simulink model "P4p2_integral"  (R2014a)
settings: Solver=ode1  StartTime=0.0  StopTime=inf  FixedStep=0.002  RelTol=1e-3
PostLoadFcn:
  | qc_set_target_type(getConfigSet(bdroot, 'QUARC Default Target Configuration'));
values from neighbouring files (symbols this model uses):
  A_est = [0 1 0 0 0 0; 0 0 0 0 0 0; 0 0 0 1 0 0; 0 0 0 0 0 0; 0 0 0 0 0 1; k_3 0 0 0 0 0]    [P4p2_init.m]    (also in P4p2_integral_init.m = [0 1 0 0 0 0; 0 0 0 0 0 0; 0 0 0 1 0 0; P4p3_init.m = [0 1 0 0 0 0; 0 0 0 0 0 0; 0 0 0 1 0 0)
  B_est = [0 0; 0 k_1; 0 0; k_2 0;0 0; 0 0]    [P4p2_init.m]    (also in P4p2_integral_init.m; P4p3_init.m)
  C_est = [1 0 0 0 0 0; 0 0 1 0 0 0; 0 0 0 0 1 0]    [P4p2_init.m]    (also in P4p2_integral_init.m; P4p3_init.m = [0 0 1 0 0 0; 0 0 0 0 1 0])
  Joystick_gain_x = 1    [P4p2_init.m]    (also in P4p2_integral_init.m; P4p3_init.m)
  Joystick_gain_y = -1    [P4p2_init.m]    (also in P4p2_integral_init.m; P4p3_init.m)
  K = lqr(A, B, Q, R)    [P4p2_init.m]    (also in P4p2_integral_init.m = lqr(A,B,Q,R); P4p3_init.m = lqr(A,B,Q,R))
  L = (place(A_est', C_est', poles)')    [P4p2_init.m]    (also in P4p2_integral_init.m; P4p3_init.m)
  P = inv(C*(inv(B*K - A))*B)    [P4p2_init.m]    (also in P4p2_integral_init.m = [0  K(2,1); K(1,3) 0]; P4p3_init.m = [0  K(2,1); K(1,3) 0])
  v_star = 6.8    [P4p2_init.m]    (also in P4p2_integral_init.m; P4p3_init.m)
undefined symbols (not defined in the file or in its folder): HIL, qc_get_step_size
libraries: simulink_extras x7, quarc_library x4
settings Model: SimulationMode=external  ExtModeTrigDuration=5000  Creator=Rchan  LastModifiedBy=kajajs
settings SolverCC: PositivePriorityOrder=on
settings DataIOCC: SignalLoggingSaveFormat=ModelDataLogs
settings OptimizationCC: ExpressionDepthLimit=2147483647  InitFltsAndDblsToZero=on
settings DebuggingCC: SaveWithParameterizedLinksMsg=none  UnderspecifiedInitializationDetection=Classic  MultiTaskDSMMsg=warning  MultiTaskCondExecSysMsg=none  FcnCallInpInsideContextMsg=UseLocalSettings  StateNameClashWarn=warning
settings RTWCC: SystemTargetFile=quarc_win64.tlc  TemplateMakefile=quarc_default_tmf  Description=QUARC Win64 Target  ProcessScript=quarc_win64_make_rtw_hook
settings STFCustomTargetCC: CPPClassGenCompliant=on
settings GRTTargetCC: ParMdlRefBuildCompliant=off  CompOptLevelCompliant=off  CombineOutputUpdateFcns=off  MatFileLogging=off  GRTInterface=on  ExtMode=on  ExtModeMexFile=quarc_comm

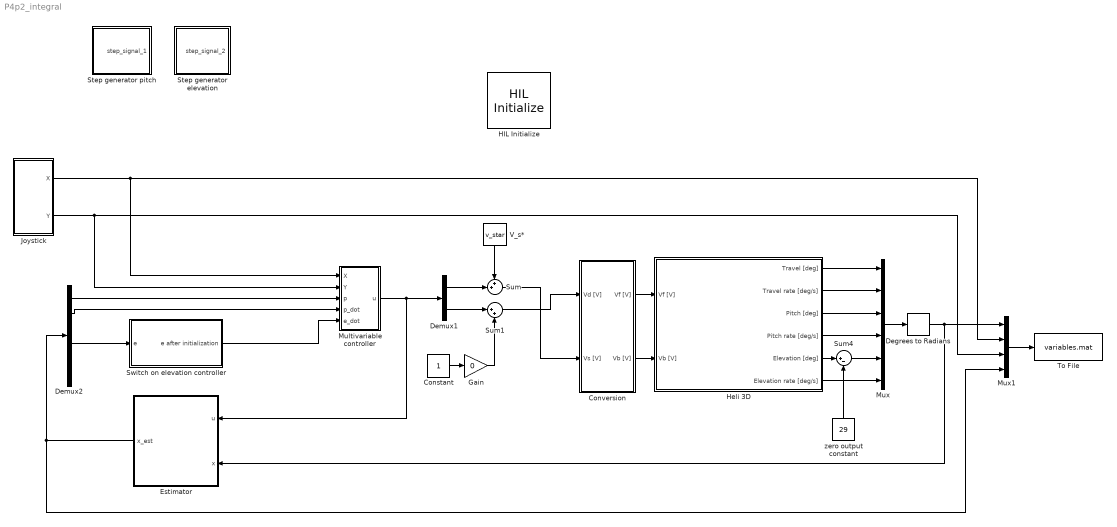
== system P4p2_integral ==
  " Switch on elevation controller" : Subsystem
  Constant : Constant
  Conversion : Subsystem
  Degrees to Radians : simulink_extras/Transformations/Degrees to Radians
  Demux1 : Demux  Outputs=2
  Demux2 : Demux  Outputs=6
  Estimator : Subsystem
  Gain : Gain  Gain=0
  HIL Initialize : quarc_library/Data Acquisition/Generic/Configuration/HIL Initialize  Priority=-99  object_name=HIL-1  board_type=q8_usb  board_number=0  board_options=update_rate=normal;decimation=1  exclusive=off  active=off  hardware_clocks=[0:2]  clock_modes=[]  initial_clock_frequencies=[]  set_clock_params_at_start=off  set_clock_params_at_switch_in=off  set_clock_frequencies_at_start=off  set_clock_frequencies_at_switch_in=off  analog_input_channels=[0:7]  analog_input_maximums=10  analog_input_minimums=-10  set_analog_input_params_at_start=on  set_analog_input_params_at_switch_in=off  analog_output_channels=[0:7]  analog_output_maximums=10  analog_output_minimums=-10  initial_analog_outputs=[0]  final_analog_outputs=[0]  watchdog_analog_outputs=0  set_analog_output_params_at_start=on  set_analog_output_params_at_switch_in=off  set_analog_outputs_at_start=on  set_analog_outputs_at_switch_in=off  set_analog_outputs_at_terminate=on  set_analog_outputs_at_switch_out=off  set_analog_outputs_on_watchdog=off  digital_input_channels=[]  digital_output_channels=[]  digital_output_configuration=[]  initial_digital_outputs=[1]  final_digital_outputs=[1]  watchdog_digital_outputs=[1]  set_digital_output_params_at_start=off  set_digital_output_params_at_switch_in=off  set_digital_outputs_at_start=on  set_digital_outputs_at_switch_in=off  set_digital_outputs_at_terminate=on  set_digital_outputs_at_switch_out=off  set_digital_outputs_on_watchdog=off  encoder_channels=[0:7]  quadrature=[4]  encoder_filter_frequency=[]  initial_encoder_counts=[0]  set_encoder_params_at_start=on  set_encoder_params_at_switch_in=off  set_encoder_counts_at_start=on  set_encoder_counts_at_switch_in=off  pwm_channels=[0:7]  pwm_modes=0  pwm_frequency=99.532799999999995e6/4095  pwm_configuration=[0]  pwm_alignment=[0]  pwm_polarity=[1]  pwm_leading_deadband=[0]  pwm_trailing_deadband=[0]  initial_pwm_outputs=[0]  final_pwm_outputs=[0]  watchdog_pwm_outputs=[0]  set_pwm_params_at_start=on  set_pwm_params_at_switch_in=off  set_pwm_outputs_at_start=on  set_pwm_outputs_at_switch_in=off  set_pwm_outputs_at_terminate=on  set_pwm_outputs_at_switch_out=off  set_pwm_outputs_on_watchdog=off  other_output_channels=[]  initial_other_outputs=[]  final_other_outputs=[]  watchdog_other_outputs=[]  set_other_outputs_at_start=off  set_other_outputs_at_switch_in=off  set_other_outputs_at_terminate=off  set_other_outputs_at_switch_out=off  set_other_outputs_on_watchdog=off
  Heli 3D : Subsystem
  Joystick : Subsystem
  "Multivariable controller " : Subsystem
  Mux : Mux  Inputs=6
  Mux1 : Mux
  Step generator elevation : Subsystem
  Step generator pitch : Subsystem
  Sum : Sum  Inputs=++|
  Sum1 : Sum  Inputs=|++
  Sum4 : Sum  Inputs=|+-
  To File : ToFile  Filename=variables.mat  MatrixName=variables
  "V_s*    " : Constant  Value=v_star
  zero output constant : Constant  Value=29
  wires:
  Conversion/2(Vb [V]) -> Heli 3D/2(Vb [V])
  Conversion/1(Vf [V]) -> Heli 3D/1(Vf [V])
  Heli 3D/1(Travel [deg]) -> Mux/1
  Heli 3D/2(Travel rate [deg/s]) -> Mux/2
  Heli 3D/4(Pitch rate [deg/s]) -> Mux/4
  Heli 3D/6(Elevation rate [deg/s]) -> Mux/6
  "Multivariable controller "/1(u) -> Estimator/1(u), Demux1/1
  Mux/1 -> Degrees to Radians/1
  Degrees to Radians/1 -> Mux1/1, Estimator/2(x)
  Sum/1 -> Conversion/2(Vs [V])
  Mux1/1 -> To File/1
  Demux1/2 -> Sum1/1
  Sum1/1 -> Conversion/1(Vd [V])
  Constant/1 -> Gain/1
  Gain/1 -> Sum1/2
  Joystick/1(X) -> Mux1/2, "Multivariable controller "/1(X)
  Joystick/2(Y) -> Mux1/3, "Multivariable controller "/2(Y)
  Demux1/1 -> Sum/2
  Heli 3D/5(Elevation [deg]) -> Sum4/1
  Sum4/1 -> Mux/5
  zero output constant/1 -> Sum4/2
  Heli 3D/3(Pitch [deg]) -> Mux/3
  "V_s*    "/1 -> Sum/1
  Estimator/1(x_est) -> Mux1/4, Demux2/1
  " Switch on elevation controller"/1("e after initialization ") -> "Multivariable controller "/5(e_dot)
  Demux2/4 -> " Switch on elevation controller"/1(e)
  Demux2/1 -> "Multivariable controller "/3(p)
  Demux2/2 -> "Multivariable controller "/4(p_dot)

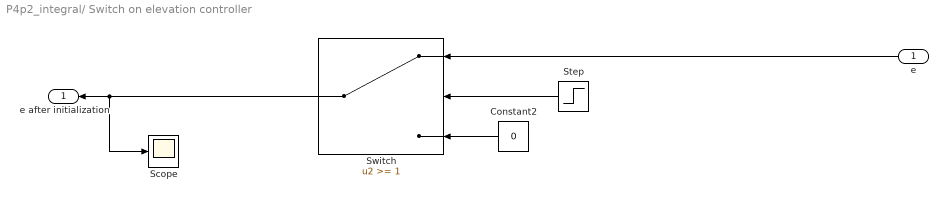
== system P4p2_integral/ Switch on elevation controller ==
  e : Inport
  Constant2 : Constant  Value=0
  Scope : Scope
      settings: YMin=-2.25  YMax=2
  Step : Step  Time=5  SampleTime=0
  Switch : Switch  Threshold=1
  "e after initialization " : Outport
  wires:
  Switch/1 -> Scope/1, "e after initialization "/1
  Constant2/1 -> Switch/3
  e/1 -> Switch/1
  Step/1 -> Switch/2

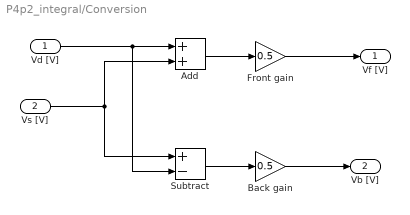
== system P4p2_integral/Conversion ==
  Vd [V] : Inport
  Vs [V] : Inport  Port=2
  Add : Sum
  Back gain : Gain  Gain=0.5
  Front gain : Gain  Gain=0.5
  Subtract : Sum  Inputs=+-
  Vf [V] : Outport
  Vb [V] : Outport  Port=2
  wires:
  Vd [V]/1 -> Subtract/2, Add/1
  Vs [V]/1 -> Subtract/1, Add/2
  Subtract/1 -> Back gain/1
  Back gain/1 -> Vb [V]/1
  Add/1 -> Front gain/1
  Front gain/1 -> Vf [V]/1

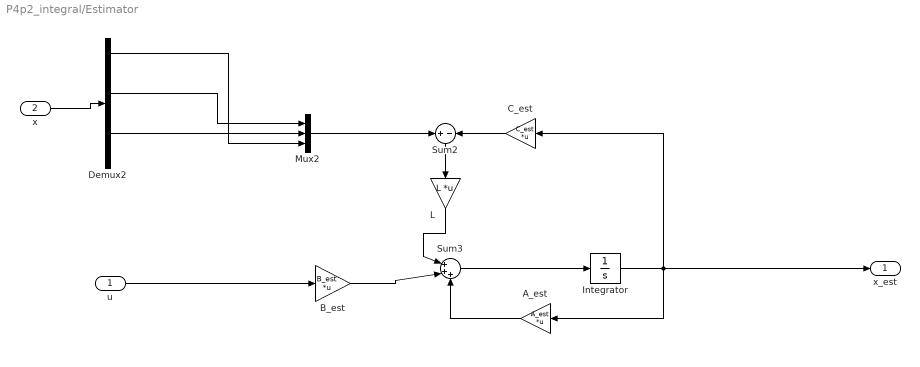
== system P4p2_integral/Estimator ==
  u : Inport
  x : Inport  Port=2
  A_est : Gain  Gain=A_est  Multiplication=Matrix(K*u)
  B_est : Gain  Gain=B_est  Multiplication=Matrix(K*u)
  C_est : Gain  Gain=C_est  Multiplication=Matrix(K*u)
  Demux2 : Demux  Outputs=6
  Integrator : Integrator
  L : Gain  Gain=L  Multiplication=Matrix(K*u)
  Mux2 : Mux  Inputs=3
  Sum2 : Sum  Inputs=+|-
  Sum3 : Sum  Inputs=|+++
  x_est : Outport
  wires:
  Demux2/5 -> Mux2/2
  Sum3/1 -> Integrator/1
  Sum2/1 -> L/1
  A_est/1 -> Sum3/3
  Demux2/3 -> Mux2/1
  Integrator/1 -> x_est/1, C_est/1, A_est/1
  B_est/1 -> Sum3/2
  Mux2/1 -> Sum2/1
  L/1 -> Sum3/1
  C_est/1 -> Sum2/2
  Demux2/1 -> Mux2/3
  u/1 -> B_est/1
  x/1 -> Demux2/1

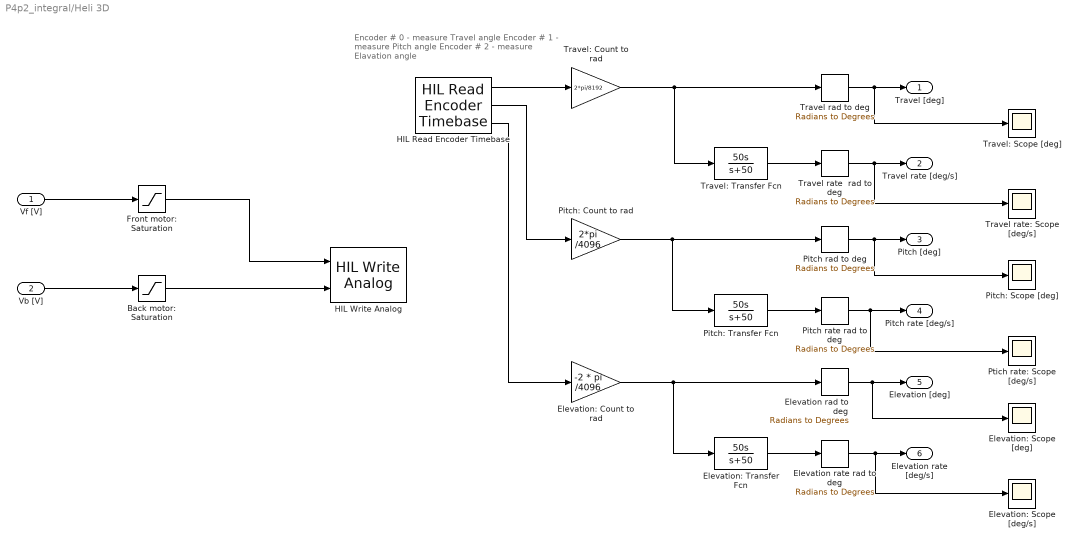
== system P4p2_integral/Heli 3D ==
  note: Encoder # 0 - measure Travel angle
      | Encoder # 1 - measure Pitch angle
      | Encoder # 2 - measure Elavation angle
  Vf [V] : Inport
  Vb [V] : Inport  Port=2
  Back motor: Saturation : Saturate  UpperLimit=5  LowerLimit=-5
  Elevation rad to deg : simulink_extras/Transformations/Radians to Degrees
  Elevation rate rad to deg : simulink_extras/Transformations/Radians to Degrees
  Elevation: Count to rad : Gain  Gain=-2 * pi /4096
  Elevation: Scope [deg/s] : Scope
      settings: YMin=-15  YMax=15  SaveName=ScopeData13
  Elevation: Scope [deg] : Scope
      settings: YMin=-15  YMax=15  SaveName=ScopeData12
  Elevation: Transfer Fcn : TransferFcn  Numerator=[50 0]  Denominator=[1 50]
  Front motor: Saturation : Saturate  UpperLimit=5  LowerLimit=-5
  HIL Read Encoder Timebase : quarc_library/Data Acquisition/Generic/Timebases/HIL Read Encoder Timebase  object_name=HIL-1  clock=0  channels=[0:2]  samples_in_buffer=max(ceil(1/qc_get_step_size), 1)  active=on  vector_output=off  data_type_mode=Inherit via back propagation  data_type=double
  HIL Write Analog : quarc_library/Data Acquisition/Generic/Immediate I//O/HIL Write Analog  object_name=HIL-1  channels=[0:1]  sample_time=-1  active=off  vector_input=off
  Pitch rad to deg : simulink_extras/Transformations/Radians to Degrees
  Pitch rate rad to deg : simulink_extras/Transformations/Radians to Degrees
  Pitch: Count to rad : Gain  Gain=2*pi /4096
  Pitch: Scope [deg] : Scope
      settings: YMin=-15  YMax=15  SaveName=ScopeData10
  Pitch: Transfer Fcn : TransferFcn  Numerator=[50 0]  Denominator=[1 50]
  Ptich rate: Scope [deg/s] : Scope
      settings: YMin=-15  YMax=15  SaveName=ScopeData11
  Travel rad to deg : simulink_extras/Transformations/Radians to Degrees
  Travel rate  rad to deg : simulink_extras/Transformations/Radians to Degrees
  Travel rate: Scope [deg/s] : Scope
      settings: YMin=-15  YMax=15  SaveName=ScopeData9
  Travel: Count to rad : Gain  Gain=2*pi/8192
  Travel: Scope [deg] : Scope
      settings: YMin=-15  YMax=15  SaveName=ScopeData8
  Travel: Transfer Fcn : TransferFcn  Numerator=[50 0]  Denominator=[1 50]
  Travel [deg] : Outport
  Travel rate [deg/s] : Outport  Port=2
  Pitch [deg] : Outport  Port=3
  Pitch rate [deg/s] : Outport  Port=4
  Elevation [deg] : Outport  Port=5
  Elevation rate [deg/s] : Outport  Port=6
  wires:
  HIL Read Encoder Timebase/1 -> Travel: Count to rad/1
  HIL Read Encoder Timebase/2 -> Pitch: Count to rad/1
  HIL Read Encoder Timebase/3 -> Elevation: Count to rad/1
  Travel: Count to rad/1 -> Travel: Transfer Fcn/1, Travel rad to deg/1
  Travel: Transfer Fcn/1 -> Travel rate  rad to deg/1
  Pitch: Count to rad/1 -> Pitch: Transfer Fcn/1, Pitch rad to deg/1
  Pitch: Transfer Fcn/1 -> Pitch rate rad to deg/1
  Elevation: Count to rad/1 -> Elevation: Transfer Fcn/1, Elevation rad to deg/1
  Elevation: Transfer Fcn/1 -> Elevation rate rad to deg/1
  Travel rad to deg/1 -> Travel: Scope [deg]/1, Travel [deg]/1
  Travel rate  rad to deg/1 -> Travel rate: Scope [deg/s]/1, Travel rate [deg/s]/1
  Pitch rad to deg/1 -> Pitch: Scope [deg]/1, Pitch [deg]/1
  Pitch rate rad to deg/1 -> Ptich rate: Scope [deg/s]/1, Pitch rate [deg/s]/1
  Elevation rad to deg/1 -> Elevation: Scope [deg]/1, Elevation [deg]/1
  Elevation rate rad to deg/1 -> Elevation: Scope [deg/s]/1, Elevation rate [deg/s]/1
  Vf [V]/1 -> Front motor: Saturation/1
  Vb [V]/1 -> Back motor: Saturation/1
  Front motor: Saturation/1 -> HIL Write Analog/1
  Back motor: Saturation/1 -> HIL Write Analog/2

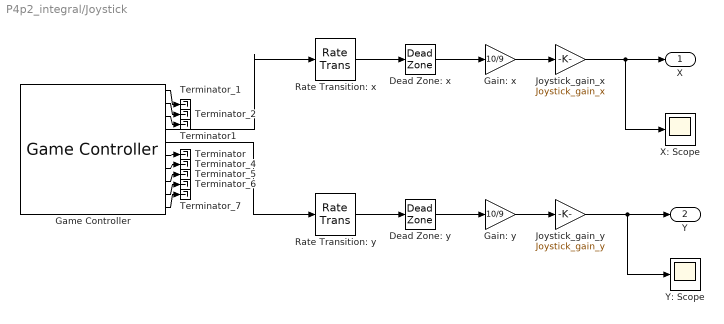
== system P4p2_integral/Joystick ==
  Dead Zone: x : DeadZone  LowerValue=-0.1  UpperValue=0.1  SaturateOnIntegerOverflow=on
  Dead Zone: y : DeadZone  LowerValue=-0.1  UpperValue=0.1  SaturateOnIntegerOverflow=on
  Gain: x : Gain  Gain=10/9
  Gain: y : Gain  Gain=10/9
  Game Controller : quarc_library/Devices/Peripherals/Target/Game Controller  controller=1  buffer_size=12  deadzone=[]  saturation=[]  sample_time=max(qc_get_step_size, 0.01)  auto_center=off  enabled=on
  Joystick_gain_x : Gain  Gain=Joystick_gain_x
  Joystick_gain_y : Gain  Gain=Joystick_gain_y
  Rate Transition: x : RateTransition
  Rate Transition: y : RateTransition
  Terminator : Terminator
  Terminator1 : Terminator
  Terminator_{1..2,4..7} (6 alike) : Terminator
  X: Scope : Scope
      settings: YMin=-1  YMax=1  SaveName=ScopeData7
  Y: Scope : Scope
      settings: YMin=-10  YMax=10  SaveName=ScopeData5
  X : Outport
  Y : Outport  Port=2
  wires:
  Rate Transition: y/1 -> Dead Zone: y/1
  Rate Transition: x/1 -> Dead Zone: x/1
  Game Controller/5 -> Rate Transition: y/1
  Game Controller/4 -> Rate Transition: x/1
  Game Controller/1 -> Terminator_1/1
  Game Controller/2 -> Terminator_2/1
  Game Controller/7 -> Terminator_4/1
  Game Controller/8 -> Terminator_5/1
  Game Controller/9 -> Terminator_6/1
  Game Controller/10 -> Terminator_7/1
  Game Controller/3 -> Terminator1/1
  Game Controller/6 -> Terminator/1
  Dead Zone: x/1 -> Gain: x/1
  Dead Zone: y/1 -> Gain: y/1
  Gain: x/1 -> Joystick_gain_x/1
  Gain: y/1 -> Joystick_gain_y/1
  Joystick_gain_x/1 -> X/1, X: Scope/1
  Joystick_gain_y/1 -> Y: Scope/1, Y/1

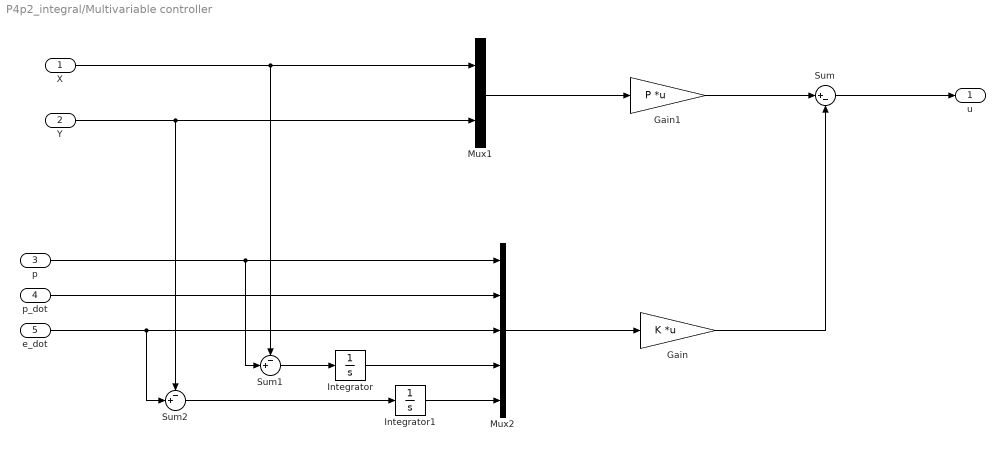
== system P4p2_integral/Multivariable controller  ==
  X : Inport
  Y : Inport  Port=2
  p : Inport  Port=3
  p_dot : Inport  Port=4
  e_dot : Inport  Port=5
  Gain : Gain  Gain=K  Multiplication=Matrix(K*u) (u vector)
  Gain1 : Gain  Gain=P  Multiplication=Matrix(K*u) (u vector)
  Integrator : Integrator
  Integrator1 : Integrator
  Mux1 : Mux  Inputs=2
  Mux2 : Mux  Inputs=5
  Sum : Sum  Inputs=|+-
  Sum1 : Sum  Inputs=-+|
  Sum2 : Sum  Inputs=-+|
  u : Outport
  wires:
  X/1 -> Mux1/1, Sum1/1
  Y/1 -> Mux1/2, Sum2/1
  Gain1/1 -> Sum/1
  Mux1/1 -> Gain1/1
  Mux2/1 -> Gain/1
  Gain/1 -> Sum/2
  Sum/1 -> u/1
  p/1 -> Sum1/2, Mux2/1
  e_dot/1 -> Mux2/3, Sum2/2
  Sum1/1 -> Integrator/1
  Sum2/1 -> Integrator1/1
  Integrator/1 -> Mux2/4
  Integrator1/1 -> Mux2/5
  p_dot/1 -> Mux2/2

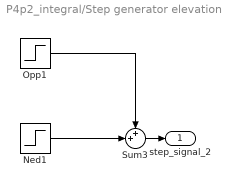
== system P4p2_integral/Step generator elevation ==
  Ned1 : Step  Time=25  After=-0.2  SampleTime=0
  Opp1 : Step  Time=22  After=0.2  SampleTime=0
  Sum3 : Sum  Inputs=++|
  step_signal_2 : Outport
  wires:
  Opp1/1 -> Sum3/1
  Ned1/1 -> Sum3/2
  Sum3/1 -> step_signal_2/1

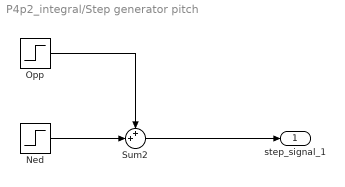
== system P4p2_integral/Step generator pitch ==
  Ned : Step  Time=17  After=-0.4  SampleTime=0
  Opp : Step  Time=10  After=0.4  SampleTime=0
  Sum2 : Sum  Inputs=++|
  step_signal_1 : Outport
  wires:
  Opp/1 -> Sum2/1
  Ned/1 -> Sum2/2
  Sum2/1 -> step_signal_1/1
